simulink model "Simulink_Arduino_PIL_v05_r2018a"  (R2018a)
settings: Solver=VariableStepAuto  StartTime=0.0  StopTime=Tsim  RelTol=1e-3
values from neighbouring files (symbols this model uses):
  Ac = [-112.5 0 0 1 0 0 0 -112.5 0 0 1 0 ... (36 elements, 6x6)]    [exitationData.mat]    (also in main_Simulink_Arduino_PIL_v05.m = [0 1 0 0 0 0; main_Simulink_Arduino_PIL_v05_v2.m = sys_ct.A; result_data.mat = [-27.8072490393 38.7615323826 -12.4282188209 -19.7589667718 )
  Bc = [1250  0; 0  1250; 0  0; 0  0; 0  0; 0  0]    [exitationData.mat]    (also in main_Simulink_Arduino_PIL_v05.m = [0 0; main_Simulink_Arduino_PIL_v05_v2.m = sys_ct.B; result_data.mat = [429.723017402  565.379444728; -795.881801648  -708.39184256)
  Cc = [0.5  0.5  0  0  0  0; 0  0  0  0  0  -1]    [exitationData.mat]    (also in main_Simulink_Arduino_PIL_v05.m = [0 1/2 0 1/2 0 0; main_Simulink_Arduino_PIL_v05_v2.m = sys_ct.C; result_data.mat = [0.284296065909  -0.589150784937  0.0969360429014  -0.011889)
  PIL = 0    [exitationData.mat]    (also in main_Simulink_Arduino_PIL_v05.m; main_Simulink_Arduino_PIL_v05_v2.m = 1; result_data.mat)
  Ts = 1/fs    (= 0.01)    [Model_2i2o.m]    (also in SystemIdentification.m = 0.001; exitationData.mat = 0.001; main_Simulink_Arduino_PIL_v05.m; main_Simulink_Arduino_PIL_v05_v2.m)
  xo = [0 0 0 0 0 0]    [exitationData.mat]    (also in main_Simulink_Arduino_PIL_v05.m = [0 0 0 0 0 0]'; main_Simulink_Arduino_PIL_v05_v2.m = [O1_dot_o, O2_dot_o, x_dot_o, O1_o, O2_o, x_o]'; result_data.mat)
undefined symbols (not defined in the file or in its folder): serial
libraries: instrumentlib x3
settings Model: EnablePacing=on  Creator=ricardo  LastModifiedBy=Ricardo
settings SFSimCC: SimUseLocalCustomCode=on
settings RTWCC: RTWUseLocalCustomCode=on

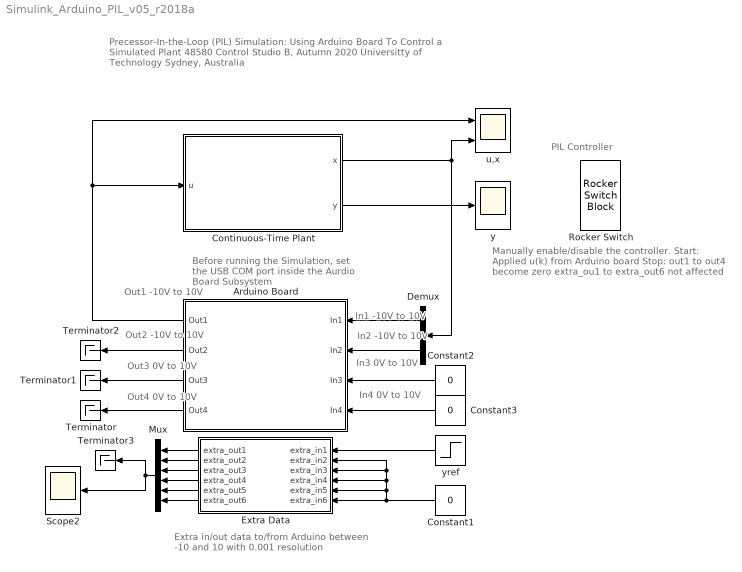
== system Simulink_Arduino_PIL_v05_r2018a ==
  note: Out1
      | -10V to 10V
  note: Precessor-In-the-Loop (PIL) Simulation:
      | Using Arduino Board To Control a Simulated Plant
      |
      | 48580 Control Studio B, Autumn 2020
      | Universitty of Technology Sydney, Australia
  note: Out2
      | -10V to 10V
  note: Out3
      | 0V to 10V
  note: Out4
      | 0V to 10V
  note: In1
      | -10V to 10V
  note: In2
      | -10V to 10V
  note: In3
      | 0V to 10V
  note: In4
      | 0V to 10V
  note: Before running the Simulation, set the USB COM port inside the Aurdio Board Subsystem
  note: PIL Controller
  note: Manually enable/disable the controller.
      | Start: Applied u(k) from Arduino board
      | Stop: out1 to out4 become zero
      | extra_ou1 to extra_out6 not affected
  note: Extra in/out data to/from Arduino between -10 and 10 with 0.001 resolution
  Arduino Board : Subsystem
      mask Display: image('UTS_MKR_Board_v031.png')
  Constant1 : Constant  Value=0
  Constant2 : Constant  Value=0
  Constant3 : Constant  Value=0
  Continuous-Time Plant : Subsystem
  Demux : Demux  Outputs=2
  Extra Data : Subsystem
  Mux : Mux  Inputs=6
  Rocker Switch : RockerSwitchBlock  LabelPosition=Hide  WebBlockId=169
      settings: Values={{'Stop', 'Start'}, [0 1]}
  Scope2 : Scope
  Terminator{,1..3} (4 alike) : Terminator
  u,x : Scope  NumInputPorts=2
  y : Scope
  yref : Step  Time=5  Before=4  After=-4  SampleTime=0
  wires:
  Continuous-Time Plant/2(y) -> y/1
  Continuous-Time Plant/1(x) -> u,x/2, Demux/1
  Demux/1 -> Arduino Board/1(In1)
  Demux/2 -> Arduino Board/2(In2)
  Arduino Board/1(Out1) -> u,x/1, Continuous-Time Plant/1(u)
  Arduino Board/2(Out2) -> Terminator2/1
  Arduino Board/3(Out3) -> Terminator1/1
  Arduino Board/4(Out4) -> Terminator/1
  Constant2/1 -> Arduino Board/3(In3)
  Constant3/1 -> Arduino Board/4(In4)
  Extra Data/1(extra_out1) -> Mux/1
  Extra Data/2(extra_out2) -> Mux/2
  Extra Data/3(extra_out3) -> Mux/3
  Extra Data/4(extra_out4) -> Mux/4
  Mux/1 -> Scope2/1, Terminator3/1
  yref/1 -> Extra Data/1(extra_in1)
  Extra Data/5(extra_out5) -> Mux/5
  Extra Data/6(extra_out6) -> Mux/6
  Constant1/1 -> Extra Data/5(extra_in5), Extra Data/2(extra_in2), Extra Data/3(extra_in3), Extra Data/4(extra_in4), Extra Data/6(extra_in6)

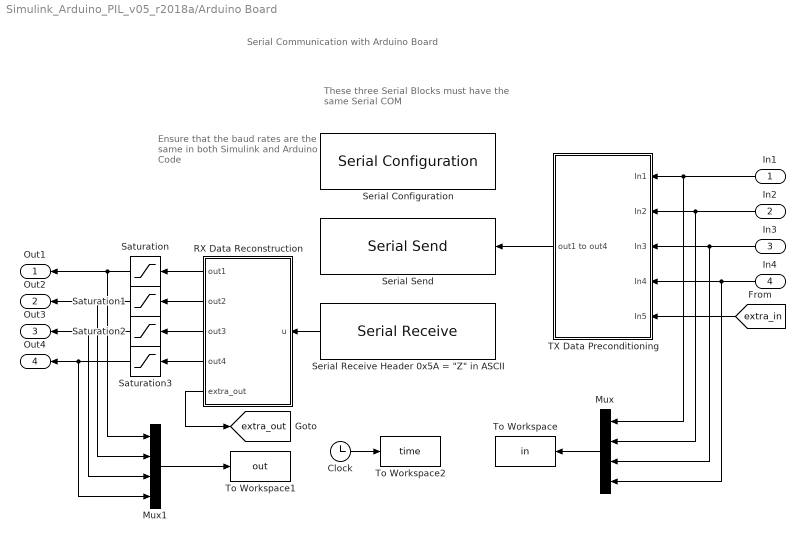
== system Simulink_Arduino_PIL_v05_r2018a/Arduino Board ==
  note: Ensure that the baud rates are the same in both Simulink and Arduino Code
  note: Serial Communication with Arduino Board
  note: These three Serial Blocks must have the same Serial COM
  In1 : Inport
  In2 : Inport  Port=2
  In3 : Inport  Port=3
  In4 : Inport  Port=4
  Clock : Clock
  Mux : Mux
  Mux1 : Mux
  RX Data Reconstruction : MATLAB Function  TreatAsAtomicUnit=on
  Saturation : Saturate  UpperLimit=10  LowerLimit=-10
  Saturation1 : Saturate  UpperLimit=10  LowerLimit=-10
  Saturation2 : Saturate  UpperLimit=10  LowerLimit=0
  Saturation3 : Saturate  UpperLimit=10  LowerLimit=0
  Serial Configuration : instrumentlib/Serial Configuration  Priority=-200000  ComPortMenu=<Please select a port...>  ComPort=/dev/cu.usbmodem141201  ObjConstructor=serial('/dev/cu.usbmodem141201');  BaudRate=115200  DataBits=8  Parity=none  StopBits=1  FlowControl=none  Timeout=0.0001  ByteOrder=LittleEndian
  "Serial Receive Header 0x5A = \"Z\" in ASCII" : instrumentlib/Serial Receive  ComPortMenu=<Please select a port...>  ComPort=/dev/cu.usbmodem141201  ObjConstructor=serial('/dev/cu.usbmodem141201');  Header=Z  Terminator=<none>  DataSize=21  DataType=uint8  EnableBlockingMode=on  ActionDataUnavailable=Output last received value  CustomValue=0  SampleTime=0.5*Ts
  Serial Send : instrumentlib/Serial Send  ComPortMenu=<Please select a port...>  ComPort=/dev/cu.usbmodem141201  ObjConstructor=serial('/dev/cu.usbmodem141201');  Terminator=<none>  EnableBlockingMode=on
  TX Data Preconditioning : Subsystem
  To Workspace : ToWorkspace  VariableName=in  SampleTime=Ts/20
  To Workspace1 : ToWorkspace  VariableName=out  SampleTime=Ts/20
  To Workspace2 : ToWorkspace  VariableName=time  SampleTime=Ts/20
  Out1 : Outport  VectorParamsAs1DForOutWhenUnconnected=off
  Out2 : Outport  Port=2  VectorParamsAs1DForOutWhenUnconnected=off
  Out3 : Outport  Port=3  VectorParamsAs1DForOutWhenUnconnected=off
  Out4 : Outport  Port=4  VectorParamsAs1DForOutWhenUnconnected=off
  tag scope: extra_out=global
  wires:
  "Serial Receive Header 0x5A = \"Z\" in ASCII"/1 -> RX Data Reconstruction/1(u)
  In1/1 -> TX Data Preconditioning/1(In1), Mux/1
  In2/1 -> TX Data Preconditioning/2(In2), Mux/2
  In3/1 -> TX Data Preconditioning/3(In3), Mux/3
  In4/1 -> TX Data Preconditioning/4(In4), Mux/4
  TX Data Preconditioning/1(out1 to out4) -> Serial Send/1
  RX Data Reconstruction/1(out1) -> Saturation/1
  RX Data Reconstruction/2(out2) -> Saturation1/1
  RX Data Reconstruction/3(out3) -> Saturation2/1
  Mux/1 -> To Workspace/1
  Mux1/1 -> To Workspace1/1
  Clock/1 -> To Workspace2/1
  Saturation/1 -> Out1/1, Mux1/1
  Saturation1/1 -> Out2/1, Mux1/2
  Saturation2/1 -> Out3/1, Mux1/3
  Saturation3/1 -> Out4/1, Mux1/4
  RX Data Reconstruction/4(out4) -> Saturation3/1
  [extra_in] -> TX Data Preconditioning/5(In5)
  RX Data Reconstruction/5(extra_out) -> [extra_out]

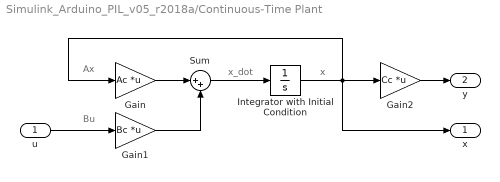
== system Simulink_Arduino_PIL_v05_r2018a/Continuous-Time Plant ==
  note: x
  note: x_dot
  note: Bu
  note: Ax
  u : Inport
  Gain : Gain  Gain=Ac  Multiplication=Matrix(K*u)
  Gain1 : Gain  Gain=Bc  Multiplication=Matrix(K*u)
  Gain2 : Gain  Gain=Cc  Multiplication=Matrix(K*u)
  Integrator with Initial Condition : Integrator  InitialCondition=xo
  Sum : Sum  Inputs=|++
  x : Outport  VectorParamsAs1DForOutWhenUnconnected=off
  y : Outport  Port=2  VectorParamsAs1DForOutWhenUnconnected=off
  wires:
  u/1 -> Gain1/1
  Gain1/1 -> Sum/2
  Sum/1 -> Integrator with Initial Condition/1
  Gain/1 -> Sum/1
  Integrator with Initial Condition/1 -> Gain2/1, x/1, Gain/1
  Gain2/1 -> y/1

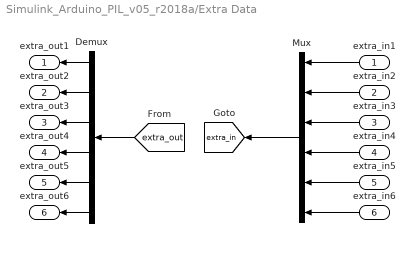
== system Simulink_Arduino_PIL_v05_r2018a/Extra Data ==
  extra_in1 : Inport
  extra_in2 : Inport  Port=2
  extra_in3 : Inport  Port=3
  extra_in4 : Inport  Port=4
  extra_in5 : Inport  Port=5
  extra_in6 : Inport  Port=6
  Demux : Demux  Outputs=6
  Mux : Mux  Inputs=6
  extra_out1 : Outport
  extra_out2 : Outport  Port=2
  extra_out3 : Outport  Port=3
  extra_out4 : Outport  Port=4
  extra_out5 : Outport  Port=5
  extra_out6 : Outport  Port=6
  tag scope: extra_in=global
  wires:
  extra_in4/1 -> Mux/4
  extra_in3/1 -> Mux/3
  extra_in2/1 -> Mux/2
  extra_in1/1 -> Mux/1
  Mux/1 -> [extra_in]
  [extra_out] -> Demux/1
  Demux/1 -> extra_out1/1
  Demux/2 -> extra_out2/1
  Demux/3 -> extra_out3/1
  Demux/4 -> extra_out4/1
  extra_in5/1 -> Mux/5
  extra_in6/1 -> Mux/6
  Demux/6 -> extra_out6/1
  Demux/5 -> extra_out5/1

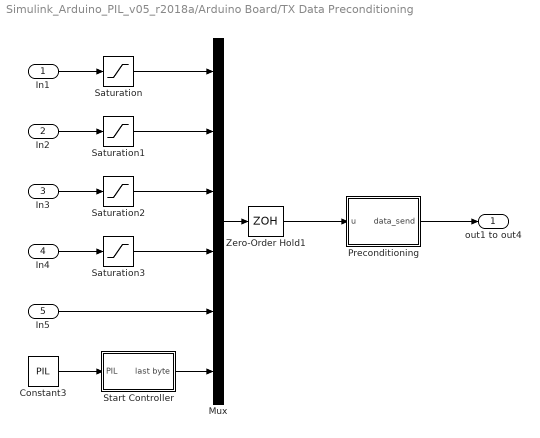
== system Simulink_Arduino_PIL_v05_r2018a/Arduino Board/TX Data Preconditioning ==
  In1 : Inport
  In2 : Inport  Port=2
  In3 : Inport  Port=3
  In4 : Inport  Port=4
  In5 : Inport  Port=5
  Constant3 : Constant  Value=PIL
  Mux : Mux  Inputs=6
  Preconditioning : MATLAB Function  TreatAsAtomicUnit=on
  Saturation : Saturate  UpperLimit=10  LowerLimit=-10
  Saturation1 : Saturate  UpperLimit=10  LowerLimit=-10
  Saturation2 : Saturate  UpperLimit=10  LowerLimit=0
  Saturation3 : Saturate  UpperLimit=10  LowerLimit=0
  Start Controller : Subsystem
  Zero-Order Hold1 : ZeroOrderHold  SampleTime=Ts
  out1 to out4 : Outport  VectorParamsAs1DForOutWhenUnconnected=off
  wires:
  In1/1 -> Saturation/1
  Preconditioning/1(data_send) -> out1 to out4/1
  Saturation3/1 -> Mux/4
  Saturation2/1 -> Mux/3
  Saturation1/1 -> Mux/2
  In2/1 -> Saturation1/1
  Mux/1 -> Zero-Order Hold1/1
  In4/1 -> Saturation3/1
  In3/1 -> Saturation2/1
  Saturation/1 -> Mux/1
  Zero-Order Hold1/1 -> Preconditioning/1(u)
  In5/1 -> Mux/5
  Constant3/1 -> Start Controller/1(PIL)
  Start Controller/1(last byte) -> Mux/6

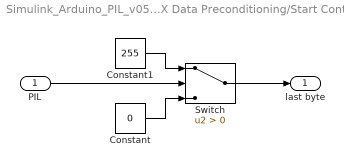
== system Simulink_Arduino_PIL_v05_r2018a/Arduino Board/TX Data Preconditioning/Start Controller ==
  PIL : Inport
  Constant : Constant  Value=0
  Constant1 : Constant  Value=255
  Switch : Switch  Criteria=u2 > Threshold
  last byte : Outport
  wires:
  Switch/1 -> last byte/1
  PIL/1 -> Switch/2
  Constant1/1 -> Switch/1
  Constant/1 -> Switch/3

== matlab function Simulink_Arduino_PIL_v05_r2018a/Arduino Board/RX Data Reconstruction ==
  data: u input; out1 output; out2 output; out3 output; out4 output; extra_out output
%% Rx Data from Arduino Board
% 
%
% 48580 Control Studio B,
% The University of Technology Sydney (UTS)
% Sydney, NSW, Australia
%
% Dr Ricardo P. Aguilera
% April 2020
%%%%%%%%%%%%%%%%%%%%%%%%%%%%%%%%%%%%%%%%%%%%%%%%%%%%%%%%%%%%%%%%%%%%%%%%%%%%

function [out1, out2, out3, out4, extra_out] = fcn(u)
N_data=10;


out=zeros(N_data,1);
extra_out=zeros(6,1);

for k=1:N_data
    %% Reconstructing out1
    MSB_uint8 = u(2*k-1); % Least Significant Bits (8 bits)
    LSB_uint8 = u(2*k);  % Most Significant Bits (8 bits)

    % Transforming MSB_uint8 in 16 bits. 
    MSB_uint16 = uint16(MSB_uint8);     %  MSB_unit16 = 00000000 | MSB_uint8 
                                                          % MSB_uint8 is stored as LSB in MSB_uint16                                             
                                                          % Therefore, it has to be shifted in 8 positions

    MSB_uint16 =bitshift(MSB_uint16,8); % MSB_unit16 = MSB_uint8 | 00000000
    out1_uint16 = MSB_uint16+ uint16(LSB_uint8);  % out1_uint16 = MSB_uint8 | LSB_uint8

    %Finally, it is transformed in its original float number
    out(k) = double(out1_uint16)*0.001-10;  
end

%% Clear out data at the beginning and when controller is not active
PIL_start = int8(0);
PIL_start = u(21);
if (PIL_start==0)
    for k=1:4
        out(k)=0;
    end
end

out1 = out(1);
out2 = out(2);
out3 = out(3);
out4 = out(4);

extra_out(1)=out(5);
extra_out(2)=out(6);
extra_out(3)=out(7);
extra_out(4)=out(8);
extra_out(5)=out(9);
extra_out(6)=out(10);

== matlab function Simulink_Arduino_PIL_v05_r2018a/Arduino Board/TX Data Preconditioning/Preconditioning ==
  data: u input; data_send output
%% Tx Data to Arduino Board
% 
%
% 48580 Control Studio B,
% The University of Technology Sydney (UTS)
% Sydney, NSW, Australia
%
% Dr Ricardo P. Aguilera
% April 2020
%%%%%%%%%%%%%%%%%%%%%%%%%%%%%%%%%%%%%%%%%%%%%%%%%%%%%%%%%%%%%%%%%%%%%%%%%%%%

function data_send = fcn(u)
N_data=10;

data_send=uint8(zeros(2*N_data+2,1));   % array of 2 bytes (2 variables of 8 bits) + Header

%Header
data_send(1)=hex2dec('AA');             %0xAA is for send data in this example

for k=1:N_data
    in = u(k);  %Input singal is between -10 to 10

    %% Data preconditioning to be transmitted as bytes

    in_pos = in+10; % to transform it in an unsigned signal between 0 to 20
    in_uint16= uint16(1000*in_pos); % Transforming it in an unsigned integer of 16 bits

    % Now, the 16 bits variable will be divided in 2 8bits variable.
    % in1_uint16 = MSB_uint8 | LSB_uint8
    % 255(dec) = 00000000|11111111 (16 bits)
    LSB_uint8  = uint8(bitand(in_uint16,255));   %Extraxting Least Significant Bits (8 bits)
    MSB_uint8 = uint8(bitshift(in_uint16,-8));    %Extraxting Most Significant Bits (8 bits)

    % Data is now put in an byte array to be transmitted
    data_send(2*k)=MSB_uint8;
    data_send(2*k+1)=LSB_uint8;
end

data_send(2*(N_data+1))=u(N_data+1);
